simulink model "UnusedModels"  (R2015a)
settings: Solver=ode45  StartTime=0.0  StopTime=10.0  RelTol=1e-3
values from neighbouring files (symbols this model uses):
  car_params = Simulink_Car_params    [TV2016_parameters.m]
  energyLimitControl = Simulink_energyLimit    [TV2016_parameters.m]
  settings = Simulink_Settings    [TV2016_parameters.m]
  speedEstimation = Simulink_speedEst    [TV2016_parameters.m]
  tractionControl = Simulink_tc    [TV2016_parameters.m]
  yawRateControl = Simulink_yawRate    [TV2016_parameters.m]
undefined symbols (not defined in the file or in its folder): canChannel, Use_Estimated_velocity
libraries: canlib x44, CarMaker4SL x33, canmsglib x28, simulink x6
(part 1 of 4)
settings Model: Creator=Will  LastModifiedBy=Will

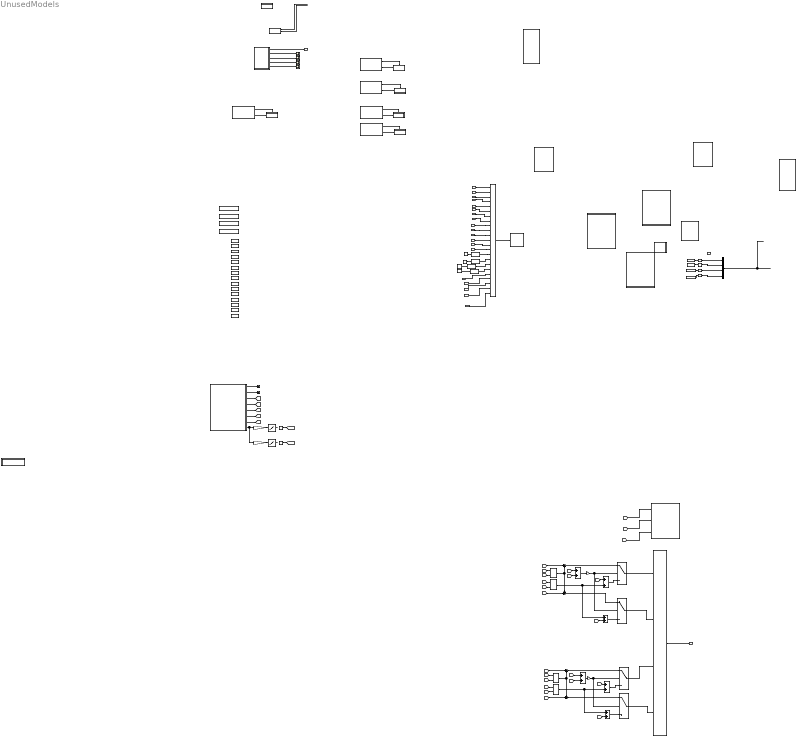
== system UnusedModels ==
  note: Tc ouput is either an increase or decrease in torque .
  "States " : Inport
  "Throttle " : Inport  Port=2
  "Brake " : Inport  Port=3
  "Steering " : Inport  Port=4
  V_x : Inport  Port=5
  V_y : Inport  Port=6
  "Fz_FL " : Inport  Port=7
  Fz_FR : Inport  Port=8
  "Fz_RL " : Inport  Port=9
  Fz_RR : Inport  Port=10
  "yawRate " : Inport  Port=11
  ay : Inport  Port=12
  ax : Inport  Port=13
  roll_angle : Inport  Port=14
  roll_rate : Inport  Port=15
  RPM_FL : Inport  Port=16
  RPM_FR : Inport  Port=17
  RPM_RL : Inport  Port=18
  RPM_RR : Inport  Port=19
  KERS_pos : Inport  Port=20
  Add{,1..5} (6 alike) : Sum
  Allocates Torque. Engineering solution : MATLAB Function  TreatAsAtomicUnit=on
  Allocates Torque. Engineering solution1 : MATLAB Function  TreatAsAtomicUnit=on
  Bus Creator : BusCreator  Inputs=23  OutDataTypeStr=Bus: SensorInputs  NonVirtualBus=on
      settings: InheritFromInputs=off
  Bus Creator1 : BusCreator  OutDataTypeStr=Bus: R_eff_i
  Bus Creator2 : BusCreator  OutDataTypeStr=Bus: Ti_lim  NonVirtualBus=on
      settings: InheritFromInputs=off
  CAN INTERFACE : Subsystem
  CAN Receive : canlib/CAN Receive  BlockHandle=13966.0022  DeviceMenu=(none)  Device=PEAK-System PCAN-USB (PCAN_USBBUS1)  ObjConstructor=canChannel('PEAK-System', 'PCAN_USBBUS1')  EnableStandardIDsFilter=off  StandardIDs=CAN_ID_INV_FL  EnableExtendedIDsFilter=off  ExtendedIDs=0  SampleTime=0.001  MsgsPerTimestep=1  StdIDsCombo=Allow only  ExtIDsCombo=Allow all  InternalFilterUpdateStatus=on
  CAN Receive1 : canlib/CAN Receive  BlockHandle=13967.002  DeviceMenu=(none)  Device=PEAK-System PCAN-USB (PCAN_USBBUS1)  ObjConstructor=canChannel('PEAK-System', 'PCAN_USBBUS1')  EnableStandardIDsFilter=off  StandardIDs=CAN_ID_INV_FR  EnableExtendedIDsFilter=off  ExtendedIDs=0  SampleTime=0.001  MsgsPerTimestep=1  StdIDsCombo=Allow only  ExtIDsCombo=Allow all  InternalFilterUpdateStatus=on
  CAN Receive2 : canlib/CAN Receive  BlockHandle=13968.0031  DeviceMenu=(none)  Device=PEAK-System PCAN-USB (PCAN_USBBUS1)  ObjConstructor=canChannel('PEAK-System', 'PCAN_USBBUS1')  EnableStandardIDsFilter=off  StandardIDs=CAN_ID_INV_RL  EnableExtendedIDsFilter=off  ExtendedIDs=0  SampleTime=0.001  MsgsPerTimestep=1  StdIDsCombo=Allow only  ExtIDsCombo=Allow all  InternalFilterUpdateStatus=on
  CAN Receive3 : canlib/CAN Receive  BlockHandle=13969.0096  DeviceMenu=(none)  Device=PEAK-System PCAN-USB (PCAN_USBBUS1)  ObjConstructor=canChannel('PEAK-System', 'PCAN_USBBUS1')  EnableStandardIDsFilter=off  StandardIDs=CAN_ID_INV_RR  EnableExtendedIDsFilter=off  ExtendedIDs=0  SampleTime=0.001  MsgsPerTimestep=1  StdIDsCombo=Allow only  ExtIDsCombo=Allow all  InternalFilterUpdateStatus=on
  CAN Receive4 : canlib/CAN Receive  BlockHandle=13970.0022  DeviceMenu=(none)  Device=PEAK-System PCAN-USB (PCAN_USBBUS1)  ObjConstructor=canChannel('PEAK-System', 'PCAN_USBBUS1')  EnableStandardIDsFilter=off  StandardIDs=[31,32,33,34]  EnableExtendedIDsFilter=off  ExtendedIDs=0  SampleTime=0.001  MsgsPerTimestep=all  StdIDsCombo=Allow only  ExtIDsCombo=Block all  InternalFilterUpdateStatus=on
  CAN Transmit : canlib/CAN Transmit  BlockHandle=14013.0021  DeviceMenu=(none)  Device=PEAK-System PCAN-USB (PCAN_USBBUS1)  ObjConstructor=canChannel('PEAK-System', 'PCAN_USBBUS1')  EnablePeriodicTransmit=on  MessagePeriod=0.005
  CAN Transmit1 : canlib/CAN Transmit  BlockHandle=14014.0021  DeviceMenu=(none)  Device=PEAK-System PCAN-USB (PCAN_USBBUS1)  ObjConstructor=canChannel('PEAK-System', 'PCAN_USBBUS1')  EnablePeriodicTransmit=on  MessagePeriod=0.005
  CAN Transmit10 : canlib/CAN Transmit  BlockHandle=14015.0021  DeviceMenu=(none)  Device=PEAK-System PCAN-USB (PCAN_USBBUS1)  ObjConstructor=canChannel('PEAK-System', 'PCAN_USBBUS1')  EnablePeriodicTransmit=on  MessagePeriod=0.005
  CAN Transmit11 : canlib/CAN Transmit  BlockHandle=14016.0021  DeviceMenu=(none)  Device=PEAK-System PCAN-USB (PCAN_USBBUS1)  ObjConstructor=canChannel('PEAK-System', 'PCAN_USBBUS1')  EnablePeriodicTransmit=on  MessagePeriod=0.005
  CAN Transmit12 : canlib/CAN Transmit  BlockHandle=14019.0021  DeviceMenu=(none)  Device=PEAK-System PCAN-USB (PCAN_USBBUS1)  ObjConstructor=canChannel('PEAK-System', 'PCAN_USBBUS1')  EnablePeriodicTransmit=on  MessagePeriod=0.005
  CAN Transmit13 : canlib/CAN Transmit  BlockHandle=14020.0021  DeviceMenu=(none)  Device=PEAK-System PCAN-USB (PCAN_USBBUS1)  ObjConstructor=canChannel('PEAK-System', 'PCAN_USBBUS1')  EnablePeriodicTransmit=on  MessagePeriod=0.005
  CAN Transmit14 : canlib/CAN Transmit  BlockHandle=14037.0066  DeviceMenu=(none)  Device=PEAK-System PCAN-USB (PCAN_USBBUS1)  ObjConstructor=canChannel('PEAK-System', 'PCAN_USBBUS1')  EnablePeriodicTransmit=on  MessagePeriod=0.005
  CAN Transmit15 : canlib/CAN Transmit  BlockHandle=14045.0049  DeviceMenu=(none)  Device=PEAK-System PCAN-USB (PCAN_USBBUS1)  ObjConstructor=canChannel('PEAK-System', 'PCAN_USBBUS1')  EnablePeriodicTransmit=on  MessagePeriod=0.005
  CAN Transmit16 : canlib/CAN Transmit  BlockHandle=14046.005  DeviceMenu=(none)  Device=PEAK-System PCAN-USB (PCAN_USBBUS1)  ObjConstructor=canChannel('PEAK-System', 'PCAN_USBBUS1')  EnablePeriodicTransmit=on  MessagePeriod=0.005
  CAN Transmit17 : canlib/CAN Transmit  BlockHandle=14047.0042  DeviceMenu=(none)  Device=PEAK-System PCAN-USB (PCAN_USBBUS1)  ObjConstructor=canChannel('PEAK-System', 'PCAN_USBBUS1')  EnablePeriodicTransmit=on  MessagePeriod=0.005
  CAN Transmit18 : canlib/CAN Transmit  BlockHandle=14048.0045  DeviceMenu=(none)  Device=PEAK-System PCAN-USB (PCAN_USBBUS1)  ObjConstructor=canChannel('PEAK-System', 'PCAN_USBBUS1')  EnablePeriodicTransmit=on  MessagePeriod=0.005
  CAN Transmit19 : canlib/CAN Transmit  BlockHandle=14206.007  DeviceMenu=(none)  Device=PEAK-System PCAN-USB (PCAN_USBBUS1)  ObjConstructor=canChannel('PEAK-System', 'PCAN_USBBUS1')  EnablePeriodicTransmit=on  MessagePeriod=0.005
  CAN Transmit3 : canlib/CAN Transmit  BlockHandle=14207.0072  DeviceMenu=(none)  Device=PEAK-System PCAN-USB (PCAN_USBBUS1)  ObjConstructor=canChannel('PEAK-System', 'PCAN_USBBUS1')  EnablePeriodicTransmit=on  MessagePeriod=0.005
  CAN Transmit4 : canlib/CAN Transmit  BlockHandle=14208.0072  DeviceMenu=(none)  Device=PEAK-System PCAN-USB (PCAN_USBBUS1)  ObjConstructor=canChannel('PEAK-System', 'PCAN_USBBUS1')  EnablePeriodicTransmit=on  MessagePeriod=0.005
  CAN Transmit5 : canlib/CAN Transmit  BlockHandle=14314.0065  DeviceMenu=(none)  Device=PEAK-System PCAN-USB (PCAN_USBBUS1)  ObjConstructor=canChannel('PEAK-System', 'PCAN_USBBUS1')  EnablePeriodicTransmit=on  MessagePeriod=0.005
  CAN Transmit6 : canlib/CAN Transmit  BlockHandle=14316.0067  DeviceMenu=(none)  Device=PEAK-System PCAN-USB (PCAN_USBBUS1)  ObjConstructor=canChannel('PEAK-System', 'PCAN_USBBUS1')  EnablePeriodicTransmit=off  MessagePeriod=0.005
  CAN Transmit7 : canlib/CAN Transmit  BlockHandle=14318.0065  DeviceMenu=(none)  Device=PEAK-System PCAN-USB (PCAN_USBBUS1)  ObjConstructor=canChannel('PEAK-System', 'PCAN_USBBUS1')  EnablePeriodicTransmit=on  MessagePeriod=0.005
  CAN Transmit8 : canlib/CAN Transmit  BlockHandle=14320.0065  DeviceMenu=(none)  Device=PEAK-System PCAN-USB (PCAN_USBBUS1)  ObjConstructor=canChannel('PEAK-System', 'PCAN_USBBUS1')  EnablePeriodicTransmit=on  MessagePeriod=0.005
  CAN Transmit9 : canlib/CAN Transmit  BlockHandle=14345.005  DeviceMenu=(none)  Device=PEAK-System PCAN-USB (PCAN_USBBUS1)  ObjConstructor=canChannel('PEAK-System', 'PCAN_USBBUS1')  EnablePeriodicTransmit=on  MessagePeriod=0.005
  Coasting KERS at 0 torque request : Subsystem
  Constant : Constant  Value=tractionControl.Kp
  Constant{1..4} (4 alike) : Constant
  Constant5 : Constant  Value=tractionControl.Ki
  Data Type Conversion{,1..6,12} (8 alike) : DataTypeConversion  OutDataTypeStr=single
  Energy limit Torque Reduction Controller : Subsystem
  "Estimations " : Subsystem  SystemSampleTime=settings.control_system_sample_time
  Function-Call Subsystem : Subsystem  TreatAsAtomicUnit=on
  Function-Call Subsystem1 : Subsystem  TreatAsAtomicUnit=on
  Function-Call Subsystem2 : Subsystem  TreatAsAtomicUnit=on
  Function-Call Subsystem3 : Subsystem  TreatAsAtomicUnit=on
  Function-Call Subsystem4 : Subsystem  TreatAsAtomicUnit=on
  FzCalcRaw : Scope
      settings: ShowLegends=on  TimeRange=0.5129057337220599  YMin=982.0067255187187  YMax=982.99982331966  SaveName=ScopeData4
  FzEstCoupledKalmanFilters : MATLAB Function  TreatAsAtomicUnit=on
  Fz_Estimation : Subsystem  TreatAsAtomicUnit=on
  Gain : Gain  Gain=single(3.6)
  Gain1 : Gain  Gain=-1
  Gain2 : Gain  Gain=single(3.6)
  Gain3 : Gain  Gain=-1
  Ki Loopup : Lookup_n-D  NumberOfTableDimensions=1  BreakpointsForDimension1=[0 10]  Table="[tractionControl.Ki_start  tractionControl.Ki_end]*tractionControl.Ki_scaling"  ExtrapMethod=Clip  UseLastTableValue=on  InternalRulePriority=Speed  RndMeth=Simplest  InputSameDT=on
  Kp Lookup : Lookup_n-D  NumberOfTableDimensions=1  BreakpointsForDimension1="[0  10]"  Table="[tractionControl.Kp_start  tractionControl.Kp_end]*tractionControl.Kp_scaling"  ExtrapMethod=Clip  UseLastTableValue=on  InternalRulePriority=Speed  RndMeth=Simplest  InputSameDT=on
  MATLAB Function : MATLAB Function  TreatAsAtomicUnit=on
  Min : MinMax  Inputs=2
  Min1 : MinMax  Function=max  Inputs=2
  Min4 : MinMax  Inputs=2
  Min5 : MinMax  Function=max  Inputs=2
  Read CM Dict10 : CarMaker4SL/Read CM Dict  xname=Car.WFR.Radius  xsync=off
  Read CM Dict11 : CarMaker4SL/Read CM Dict  xname=Car.WRR.Radius  xsync=off
  Read CM Dict12 : CarMaker4SL/Read CM Dict  xname=Car.WRL.Radius  xsync=off
  Read CM Dict9 : CarMaker4SL/Read CM Dict  xname=Car.WFL.Radius  xsync=off
  SimpleTv : Subsystem
  Slip rate Both3 : Subsystem
  Slip rate Both6 : Subsystem
  Slip rate FL : Subsystem
  Slip rate FL1 : Subsystem
  Slip ratio : MATLAB Function  TreatAsAtomicUnit=on
  Sum : Sum  Inputs=|++
  Sum1 : Sum  Inputs=++|
  Sum2 : Sum  Inputs=|++
  Sum4 : Sum  Inputs=++|
  Switch : Switch  Criteria=u2 > Threshold
  Switch1 : Switch  Criteria=u2 > Threshold  Threshold=0.0001
  Switch4 : Switch  Criteria=u2 > Threshold
  Switch5 : Switch  Criteria=u2 > Threshold
  Terminator : Terminator
  Terminator1 : Terminator
  "deltaFz " : Scope
      settings: ShowLegends=on  TimeRange=10  YMin=-650  YMax=50  SaveName=ScopeData5
  lateral : Scope
      settings: ShowLegends=on  TimeRange=1.971383147853736  YMin=574.5308310991956  YMax=1245.308310991957  SaveName=ScopeData8
  speedEstimate : Subsystem  TreatAsAtomicUnit=on
  vertialest : Scope
      settings: ShowLegends=on  TimeRange=2.029755579171094  YMin=-50  YMax=950  SaveName=ScopeData10
  Ti_SR : Outport
  Fz_Kalman_est : Outport  Port=2
  tag scope: SR_RL=global, SR_RR=global
  wires:
  Read CM Dict9/1 -> Data Type Conversion/1
  Read CM Dict11/1 -> Data Type Conversion2/1
  Read CM Dict12/1 -> Data Type Conversion3/1
  Read CM Dict10/1 -> Data Type Conversion1/1
  Data Type Conversion3/1 -> Bus Creator1/4  "R_RL"
  Data Type Conversion1/1 -> Bus Creator1/2  "R_FR"
  Data Type Conversion2/1 -> Bus Creator1/3  "R_RR"
  Data Type Conversion/1 -> Bus Creator1/1  "R_FL"
  Bus Creator1/1 -> ?
  "Brake "/1 -> Bus Creator/9  "Input_brake"
  "Steering "/1 -> Bus Creator/10  "Input_steering"
  Fz_RR/1 -> Bus Creator/5  "Input_Fz_RR"
  "Fz_RL "/1 -> Bus Creator/4  "Input_Fz_RL"
  "Fz_FL "/1 -> Bus Creator/2  "Input_Fz_FL"
  Fz_FR/1 -> Bus Creator/3  "Input_Fz_FR"
  V_y/1 -> Bus Creator/7  "V_y"
  V_x/1 -> Bus Creator/6  "V_x"
  "yawRate "/1 -> Bus Creator/1  "r"
  "Throttle "/1 -> Bus Creator/8  "Input_throttle"
  ay/1 -> Bus Creator/11  "ay"
  ax/1 -> Bus Creator/12  "ax"
  roll_angle/1 -> Bus Creator/13  "roll_angle"
  roll_rate/1 -> Bus Creator/14  "roll_rate"
  Constant1/1 -> Data Type Conversion12/1
  Data Type Conversion12/1 -> Bus Creator/15  "d_def_FL"
  Constant2/1 -> Data Type Conversion4/1
  Data Type Conversion4/1 -> Bus Creator/16  "d_def_FR"
  Constant3/1 -> Data Type Conversion5/1
  Data Type Conversion5/1 -> Bus Creator/17  "d_def_RL"
  Constant4/1 -> Data Type Conversion6/1
  Data Type Conversion6/1 -> Bus Creator/18  "d_def_RR"
  RPM_FL/1 -> Bus Creator/19  "RPM_FL"
  RPM_FR/1 -> Bus Creator/20  "RPM_FR"
  RPM_RL/1 -> Bus Creator/21  "RPM_RL"
  RPM_RR/1 -> Bus Creator/22  "RPM_RR"
  KERS_pos/1 -> Bus Creator/23  "KERS_pos"
  Bus Creator/1 -> "Estimations "/1("SensorInputs ")
  CAN Receive/2 -> Function-Call Subsystem/1(CAN_MSG)
  CAN Receive/1 -> Function-Call Subsystem/Trigger
  CAN Receive1/2 -> Function-Call Subsystem1/1(CAN_MSG)
  CAN Receive1/1 -> Function-Call Subsystem1/Trigger
  CAN Receive2/2 -> Function-Call Subsystem2/1(CAN_MSG)
  CAN Receive2/1 -> Function-Call Subsystem2/Trigger
  CAN Receive3/2 -> Function-Call Subsystem3/1(CAN_MSG)
  CAN Receive3/1 -> Function-Call Subsystem3/Trigger
  CAN Receive4/2 -> Function-Call Subsystem4/1(CAN_MSG)
  CAN Receive4/1 -> Function-Call Subsystem4/Trigger
  [Ti_RR] -> Slip rate Both6/3(Ti_ref)
  [SR_ref] -> Slip rate Both6/1(SR_ref)
  [SR_RR] -> Slip rate Both6/2(SR)
  Add4/1 -> Gain1/1
  Min/1 -> Sum1/1, Sum/2
  [Ti_FR] -> Sum1/2  "FR"
  Min1/1 -> Add1/1, Add/2
  Add1/1 -> Switch1/3
  [Ti_FL] -> Sum/1
  [Ti_FL] -> Add/1
  Add/1 -> Switch/3
  [TC_FL] -> Min/1
  [TC_FR] -> Min/2
  [TC_FR] -> Min1/2
  [TC_FL] -> Min1/1
  [Ti_FR] -> Add1/2
  [TC_FR] -> Add4/2
  [TC_FL] -> Add4/1
  Switch1/1 -> Bus Creator2/2  "FR"
  Switch/1 -> Bus Creator2/1  "FL"
  Gain3/1 -> Switch5/2, Switch4/2
  Min4/1 -> Sum4/1, Sum2/2
  Sum2/1 -> Switch4/1
  [Ti_RR] -> Sum4/2  "FR"
  Sum4/1 -> Switch5/1
  Min5/1 -> Add3/1, Add2/2
  Add3/1 -> Switch5/3
  [Ti_RL] -> Sum2/1
  [Ti_RL] -> Add2/1
  Add2/1 -> Switch4/3
  [TC_RL] -> Min4/1
  [TC_RR] -> Min4/2
  [TC_RR] -> Min5/2
  [TC_RL] -> Min5/1
  [Ti_RR] -> Add3/2
  [TC_RR] -> Add5/2
  [TC_RL] -> Add5/1
  Switch5/1 -> Bus Creator2/4  "RR"
  Switch4/1 -> Bus Creator2/3  "RL"
  Bus Creator2/1 -> Ti_SR/1
  Gain1/1 -> Switch1/2, Switch/2
  Add5/1 -> Gain3/1
  Sum/1 -> Switch/1
  Sum1/1 -> Switch1/1
  Slip ratio/3(SR_ref) -> [SR_ref]
  Slip ratio/4(SR_FL) -> [SR_FL]
  Slip ratio/5(SR_FR) -> [SR_FR]
  Slip ratio/6(SR_RL) -> [SR_RL]
  Slip ratio/7(SR_RR) -> [SR_RR]
  Slip ratio/2(SR_Ki) -> Terminator1/1
  Slip ratio/1(SR_Kp) -> Terminator/1
  Slip ratio/8(speed) -> Gain/1, Gain2/1
  Kp Lookup/1 -> ?
  Ki Loopup/1 -> ?
  Gain/1 -> Kp Lookup/1
  Gain2/1 -> Ki Loopup/1
  Constant5/1 -> [SR_Ki]
  Constant/1 -> [SR_Kp]
  FzEstCoupledKalmanFilters/2(x_out) -> lateral/1
  FzEstCoupledKalmanFilters/3(xv_out) -> vertialest/1
  FzEstCoupledKalmanFilters/4(FZ) -> FzCalcRaw/1
  FzEstCoupledKalmanFilters/5(delta_Fzl) -> "deltaFz "/1
  FzEstCoupledKalmanFilters/1(normalForces) -> Fz_Kalman_est/1
  ? -> Coasting KERS at 0 torque request/1(states)
  Coasting KERS at 0 torque request/1(active) -> ?
  Coasting KERS at 0 torque request/2(Ti_coast) -> ?

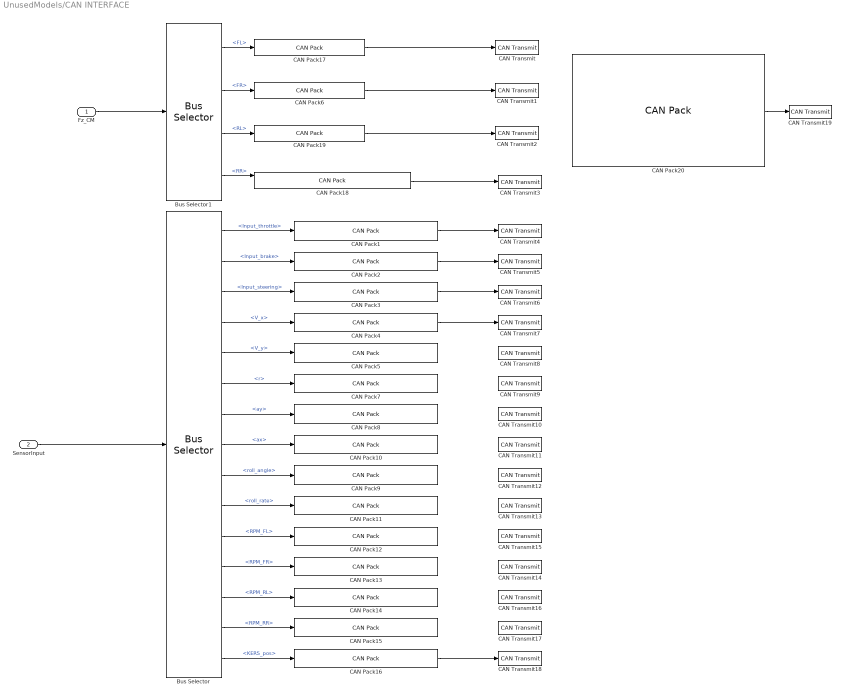
== system UnusedModels/CAN INTERFACE ==
  Fz_CM : Inport
  SensorInput : Inport  Port=2
  Bus Selector : BusSelector  OutputSignals=Input_throttle,Input_brake,Input_steering,V_x,V_y,r,ay,ax,roll_angle,roll_rate,RPM_FL,RPM_FR,RPM_RL,RPM_RR,KERS_pos
  Bus Selector1 : BusSelector  OutputSignals=FL,FR,RL,RR
  CAN Pack1 : canmsglib/CAN Pack  MsgList=(none)  MsgName=gas  MsgIDType=Standard (11-bit identifier)  MsgIdentifier=CAN_ID_GAS  MsgLength=8  SignalInfo=gas$0$32$1$3$1$0$1$0$-Inf$Inf$#  NSignals=1  StartBits=str2num('[int32(0)]')  SignalSizes=str2num('[int32(32)]')  ByteOrders=str2num('[int32(1)]')  DataTypes=str2num('[int32(3)]')  MultiplexTypes=str2num('[int32(1)]')  MultiplexValues=str2num('[double(0)]')  Factors=str2num('[double(1)]')  Offsets=str2num('[double(0)]')  Minimums=str2num('[double(-Inf)]')  Maximums=str2num('[double(Inf)]')  Remote=off
      settings: DataFormat=manually specified signals
  CAN Pack10 : canmsglib/CAN Pack  MsgList=(none)  MsgName=ax  MsgIDType=Standard (11-bit identifier)  MsgIdentifier=CAN_ID_AX  MsgLength=4  SignalInfo=ax$0$32$1$3$1$0$1$0$-Inf$Inf$#  NSignals=1  StartBits=str2num('[int32(0)]')  SignalSizes=str2num('[int32(32)]')  ByteOrders=str2num('[int32(1)]')  DataTypes=str2num('[int32(3)]')  MultiplexTypes=str2num('[int32(1)]')  MultiplexValues=str2num('[double(0)]')  Factors=str2num('[double(1)]')  Offsets=str2num('[double(0)]')  Minimums=str2num('[double(-Inf)]')  Maximums=str2num('[double(Inf)]')  Remote=off
      settings: DataFormat=manually specified signals
  CAN Pack11 : canmsglib/CAN Pack  MsgList=(none)  MsgName=roll_rate  MsgIDType=Standard (11-bit identifier)  MsgIdentifier=CAN_ID_ROLL_RATE  MsgLength=4  SignalInfo=roll_rate$0$32$1$3$1$0$1$0$-Inf$Inf$#  NSignals=1  StartBits=str2num('[int32(0)]')  SignalSizes=str2num('[int32(32)]')  ByteOrders=str2num('[int32(1)]')  DataTypes=str2num('[int32(3)]')  MultiplexTypes=str2num('[int32(1)]')  MultiplexValues=str2num('[double(0)]')  Factors=str2num('[double(1)]')  Offsets=str2num('[double(0)]')  Minimums=str2num('[double(-Inf)]')  Maximums=str2num('[double(Inf)]')  Remote=off
      settings: DataFormat=manually specified signals
  CAN Pack12 : canmsglib/CAN Pack  MsgList=(none)  MsgName=RPM_FL  MsgIDType=Standard (11-bit identifier)  MsgIdentifier=CAN_ID_RPM_FL  MsgLength=4  SignalInfo=RPM_FL$0$32$1$3$1$0$1$0$-Inf$Inf$#  NSignals=1  StartBits=str2num('[int32(0)]')  SignalSizes=str2num('[int32(32)]')  ByteOrders=str2num('[int32(1)]')  DataTypes=str2num('[int32(3)]')  MultiplexTypes=str2num('[int32(1)]')  MultiplexValues=str2num('[double(0)]')  Factors=str2num('[double(1)]')  Offsets=str2num('[double(0)]')  Minimums=str2num('[double(-Inf)]')  Maximums=str2num('[double(Inf)]')  Remote=off
      settings: DataFormat=manually specified signals
  CAN Pack13 : canmsglib/CAN Pack  MsgList=(none)  MsgName=RPM_FR  MsgIDType=Standard (11-bit identifier)  MsgIdentifier=CAN_ID_RPM_FR  MsgLength=4  SignalInfo=RPM_FR$0$32$1$3$1$0$1$0$-Inf$Inf$#  NSignals=1  StartBits=str2num('[int32(0)]')  SignalSizes=str2num('[int32(32)]')  ByteOrders=str2num('[int32(1)]')  DataTypes=str2num('[int32(3)]')  MultiplexTypes=str2num('[int32(1)]')  MultiplexValues=str2num('[double(0)]')  Factors=str2num('[double(1)]')  Offsets=str2num('[double(0)]')  Minimums=str2num('[double(-Inf)]')  Maximums=str2num('[double(Inf)]')  Remote=off
      settings: DataFormat=manually specified signals
  CAN Pack14 : canmsglib/CAN Pack  MsgList=(none)  MsgName=RPM_RL  MsgIDType=Standard (11-bit identifier)  MsgIdentifier=CAN_ID_RPM_RL  MsgLength=4  SignalInfo=RPM_RL$0$32$1$3$1$0$1$0$-Inf$Inf$#  NSignals=1  StartBits=str2num('[int32(0)]')  SignalSizes=str2num('[int32(32)]')  ByteOrders=str2num('[int32(1)]')  DataTypes=str2num('[int32(3)]')  MultiplexTypes=str2num('[int32(1)]')  MultiplexValues=str2num('[double(0)]')  Factors=str2num('[double(1)]')  Offsets=str2num('[double(0)]')  Minimums=str2num('[double(-Inf)]')  Maximums=str2num('[double(Inf)]')  Remote=off
      settings: DataFormat=manually specified signals
  CAN Pack15 : canmsglib/CAN Pack  MsgList=(none)  MsgName=RPM_RR  MsgIDType=Standard (11-bit identifier)  MsgIdentifier=CAN_ID_RPM_RR  MsgLength=4  SignalInfo=RPM_RR$0$32$1$3$1$0$1$0$-Inf$Inf$#  NSignals=1  StartBits=str2num('[int32(0)]')  SignalSizes=str2num('[int32(32)]')  ByteOrders=str2num('[int32(1)]')  DataTypes=str2num('[int32(3)]')  MultiplexTypes=str2num('[int32(1)]')  MultiplexValues=str2num('[double(0)]')  Factors=str2num('[double(1)]')  Offsets=str2num('[double(0)]')  Minimums=str2num('[double(-Inf)]')  Maximums=str2num('[double(Inf)]')  Remote=off
      settings: DataFormat=manually specified signals
  CAN Pack16 : canmsglib/CAN Pack  MsgList=(none)  MsgName=KERS_POS  MsgIDType=Standard (11-bit identifier)  MsgIdentifier=CAN_ID_KERS_POS  MsgLength=4  SignalInfo=KERS_POS$0$32$1$3$1$0$1$0$-Inf$Inf$#  NSignals=1  StartBits=str2num('[int32(0)]')  SignalSizes=str2num('[int32(32)]')  ByteOrders=str2num('[int32(1)]')  DataTypes=str2num('[int32(3)]')  MultiplexTypes=str2num('[int32(1)]')  MultiplexValues=str2num('[double(0)]')  Factors=str2num('[double(1)]')  Offsets=str2num('[double(0)]')  Minimums=str2num('[double(-Inf)]')  Maximums=str2num('[double(Inf)]')  Remote=off
      settings: DataFormat=manually specified signals
  CAN Pack17 : canmsglib/CAN Pack  MsgList=(none)  MsgName=Fz_FL  MsgIDType=Standard (11-bit identifier)  MsgIdentifier=CAN_ID_FZ_FL  MsgLength=4  SignalInfo=Fz_FL$0$32$1$3$1$0$1$0$-Inf$Inf$#  NSignals=1  StartBits=str2num('[int32(0)]')  SignalSizes=str2num('[int32(32)]')  ByteOrders=str2num('[int32(1)]')  DataTypes=str2num('[int32(3)]')  MultiplexTypes=str2num('[int32(1)]')  MultiplexValues=str2num('[double(0)]')  Factors=str2num('[double(1)]')  Offsets=str2num('[double(0)]')  Minimums=str2num('[double(-Inf)]')  Maximums=str2num('[double(Inf)]')  Remote=off
      settings: DataFormat=manually specified signals
  CAN Pack18 : canmsglib/CAN Pack  MsgList=(none)  MsgName=Fz_RR  MsgIDType=Standard (11-bit identifier)  MsgIdentifier=CAN_ID_FZ_RR  MsgLength=8  SignalInfo=Fz_RR$0$32$1$3$1$0$1$0$-Inf$Inf$#Signal2$32$32$1$1$1$0$1$0$-Inf$Inf$#  NSignals=2  StartBits=str2num('[int32(0);int32(32)]')  SignalSizes=str2num('[int32(32);int32(32)]')  ByteOrders=str2num('[int32(1);int32(1)]')  DataTypes=str2num('[int32(3);int32(1)]')  MultiplexTypes=str2num('[int32(1);int32(1)]')  MultiplexValues=str2num('[double(0);double(0)]')  Factors=str2num('[double(1);double(1)]')  Offsets=str2num('[double(0);double(0)]')  Minimums=str2num('[double(-Inf);double(-Inf)]')  Maximums=str2num('[double(Inf);double(Inf)]')  Remote=off
      settings: DataFormat=manually specified signals
  CAN Pack19 : canmsglib/CAN Pack  MsgList=(none)  MsgName=Fz_RL  MsgIDType=Standard (11-bit identifier)  MsgIdentifier=CAN_ID_FZ_RL  MsgLength=4  SignalInfo=Fz_RL$0$32$1$3$1$0$1$0$-Inf$Inf$#  NSignals=1  StartBits=str2num('[int32(0)]')  SignalSizes=str2num('[int32(32)]')  ByteOrders=str2num('[int32(1)]')  DataTypes=str2num('[int32(3)]')  MultiplexTypes=str2num('[int32(1)]')  MultiplexValues=str2num('[double(0)]')  Factors=str2num('[double(1)]')  Offsets=str2num('[double(0)]')  Minimums=str2num('[double(-Inf)]')  Maximums=str2num('[double(Inf)]')  Remote=off
      settings: DataFormat=manually specified signals
  CAN Pack2 : canmsglib/CAN Pack  MsgList=(none)  MsgName=brake  MsgIDType=Standard (11-bit identifier)  MsgIdentifier=CAN_ID_BRAKE  MsgLength=8  SignalInfo=brake$0$32$1$3$1$0$1$0$-Inf$Inf$#  NSignals=1  StartBits=str2num('[int32(0)]')  SignalSizes=str2num('[int32(32)]')  ByteOrders=str2num('[int32(1)]')  DataTypes=str2num('[int32(3)]')  MultiplexTypes=str2num('[int32(1)]')  MultiplexValues=str2num('[double(0)]')  Factors=str2num('[double(1)]')  Offsets=str2num('[double(0)]')  Minimums=str2num('[double(-Inf)]')  Maximums=str2num('[double(Inf)]')  Remote=off
      settings: DataFormat=manually specified signals
  CAN Pack20 : canmsglib/CAN Pack  MsgList=(none)  MsgName=Fz  MsgIDType=Standard (11-bit identifier)  MsgIdentifier=CAN_ID_FZ  MsgLength=8  SignalInfo=Fz_FL$0$16$1$2$1$0$1$0$-Inf$Inf$#Fz_FR$16$16$1$2$1$0$1$0$-Inf$Inf$#Fz_RL$32$16$1$2$1$0$1$0$-Inf$Inf$#Fz_RR$48$16$1$2$1$0$1$0$-Inf$Inf$#  NSignals=4  StartBits=str2num('[int32(0);int32(16);int32(32);int32(48)]')  SignalSizes=str2num('[int32(16);int32(16);int32(16);int32(16)]')  ByteOrders=str2num('[int32(1);int32(1);int32(1);int32(1)]')  DataTypes=str2num('[int32(2);int32(2);int32(2);int32(2)]')  MultiplexTypes=str2num('[int32(1);int32(1);int32(1);int32(1)]')  MultiplexValues=str2num('[double(0);double(0);double(0);double(0)]')  Factors=str2num('[double(1);double(1);double(1);double(1)]')  Offsets=str2num('[double(0);double(0);double(0);double(0)]')  Minimums=str2num('[double(-Inf);double(-Inf);double(-Inf);double(-Inf)]')  Maximums=str2num('[double(Inf);double(Inf);double(Inf);double(Inf)]')  Remote=off
      settings: DataFormat=manually specified signals
  CAN Pack3 : canmsglib/CAN Pack  MsgList=(none)  MsgName=steering  MsgIDType=Standard (11-bit identifier)  MsgIdentifier=CAN_ID_STEERING  MsgLength=8  SignalInfo=steering$0$32$1$3$1$0$1$0$-Inf$Inf$#  NSignals=1  StartBits=str2num('[int32(0)]')  SignalSizes=str2num('[int32(32)]')  ByteOrders=str2num('[int32(1)]')  DataTypes=str2num('[int32(3)]')  MultiplexTypes=str2num('[int32(1)]')  MultiplexValues=str2num('[double(0)]')  Factors=str2num('[double(1)]')  Offsets=str2num('[double(0)]')  Minimums=str2num('[double(-Inf)]')  Maximums=str2num('[double(Inf)]')  Remote=off
      settings: DataFormat=manually specified signals
  CAN Pack4 : canmsglib/CAN Pack  MsgList=(none)  MsgName=vx  MsgIDType=Standard (11-bit identifier)  MsgIdentifier=CAN_ID_VX  MsgLength=4  SignalInfo=vx$0$32$1$3$1$0$1$0$-Inf$Inf$#  NSignals=1  StartBits=str2num('[int32(0)]')  SignalSizes=str2num('[int32(32)]')  ByteOrders=str2num('[int32(1)]')  DataTypes=str2num('[int32(3)]')  MultiplexTypes=str2num('[int32(1)]')  MultiplexValues=str2num('[double(0)]')  Factors=str2num('[double(1)]')  Offsets=str2num('[double(0)]')  Minimums=str2num('[double(-Inf)]')  Maximums=str2num('[double(Inf)]')  Remote=off
      settings: DataFormat=manually specified signals
  CAN Pack5 : canmsglib/CAN Pack  MsgList=(none)  MsgName=vy  MsgIDType=Standard (11-bit identifier)  MsgIdentifier=CAN_ID_VY  MsgLength=4  SignalInfo=vy$0$32$1$3$1$0$1$0$-Inf$Inf$#  NSignals=1  StartBits=str2num('[int32(0)]')  SignalSizes=str2num('[int32(32)]')  ByteOrders=str2num('[int32(1)]')  DataTypes=str2num('[int32(3)]')  MultiplexTypes=str2num('[int32(1)]')  MultiplexValues=str2num('[double(0)]')  Factors=str2num('[double(1)]')  Offsets=str2num('[double(0)]')  Minimums=str2num('[double(-Inf)]')  Maximums=str2num('[double(Inf)]')  Remote=off
      settings: DataFormat=manually specified signals
  CAN Pack6 : canmsglib/CAN Pack  MsgList=(none)  MsgName=Fz_FR  MsgIDType=Standard (11-bit identifier)  MsgIdentifier=CAN_ID_FZ_FR  MsgLength=4  SignalInfo=Fz_FR$0$32$1$3$1$0$1$0$-Inf$Inf$#  NSignals=1  StartBits=str2num('[int32(0)]')  SignalSizes=str2num('[int32(32)]')  ByteOrders=str2num('[int32(1)]')  DataTypes=str2num('[int32(3)]')  MultiplexTypes=str2num('[int32(1)]')  MultiplexValues=str2num('[double(0)]')  Factors=str2num('[double(1)]')  Offsets=str2num('[double(0)]')  Minimums=str2num('[double(-Inf)]')  Maximums=str2num('[double(Inf)]')  Remote=off
      settings: DataFormat=manually specified signals
  CAN Pack7 : canmsglib/CAN Pack  MsgList=(none)  MsgName=r  MsgIDType=Standard (11-bit identifier)  MsgIdentifier=CAN_ID_YAW_RATE  MsgLength=4  SignalInfo=r$0$32$1$3$1$0$1$0$-Inf$Inf$#  NSignals=1  StartBits=str2num('[int32(0)]')  SignalSizes=str2num('[int32(32)]')  ByteOrders=str2num('[int32(1)]')  DataTypes=str2num('[int32(3)]')  MultiplexTypes=str2num('[int32(1)]')  MultiplexValues=str2num('[double(0)]')  Factors=str2num('[double(1)]')  Offsets=str2num('[double(0)]')  Minimums=str2num('[double(-Inf)]')  Maximums=str2num('[double(Inf)]')  Remote=off
      settings: DataFormat=manually specified signals
  CAN Pack8 : canmsglib/CAN Pack  MsgList=(none)  MsgName=ay  MsgIDType=Standard (11-bit identifier)  MsgIdentifier=CAN_ID_AY  MsgLength=4  SignalInfo=ay$0$32$1$3$1$0$1$0$-Inf$Inf$#  NSignals=1  StartBits=str2num('[int32(0)]')  SignalSizes=str2num('[int32(32)]')  ByteOrders=str2num('[int32(1)]')  DataTypes=str2num('[int32(3)]')  MultiplexTypes=str2num('[int32(1)]')  MultiplexValues=str2num('[double(0)]')  Factors=str2num('[double(1)]')  Offsets=str2num('[double(0)]')  Minimums=str2num('[double(-Inf)]')  Maximums=str2num('[double(Inf)]')  Remote=off
      settings: DataFormat=manually specified signals
  CAN Pack9 : canmsglib/CAN Pack  MsgList=(none)  MsgName=roll_angle  MsgIDType=Standard (11-bit identifier)  MsgIdentifier=CAN_ID_ROLL_ANGLE  MsgLength=4  SignalInfo=roll_angle$0$32$1$3$1$0$1$0$-Inf$Inf$#  NSignals=1  StartBits=str2num('[int32(0)]')  SignalSizes=str2num('[int32(32)]')  ByteOrders=str2num('[int32(1)]')  DataTypes=str2num('[int32(3)]')  MultiplexTypes=str2num('[int32(1)]')  MultiplexValues=str2num('[double(0)]')  Factors=str2num('[double(1)]')  Offsets=str2num('[double(0)]')  Minimums=str2num('[double(-Inf)]')  Maximums=str2num('[double(Inf)]')  Remote=off
      settings: DataFormat=manually specified signals
  CAN Transmit : canlib/CAN Transmit  BlockHandle=35.0001  DeviceMenu=PEAK-System PCAN-USB (PCAN_USBBUS1)  Device=PEAK-System PCAN-USB (PCAN_USBBUS1)  ObjConstructor=canChannel('PEAK-System', 'PCAN_USBBUS1')  EnablePeriodicTransmit=on  MessagePeriod=0.005
  CAN Transmit1 : canlib/CAN Transmit  BlockHandle=4653.0004  DeviceMenu=PEAK-System PCAN-USB (PCAN_USBBUS1)  Device=PEAK-System PCAN-USB (PCAN_USBBUS1)  ObjConstructor=canChannel('PEAK-System', 'PCAN_USBBUS1')  EnablePeriodicTransmit=on  MessagePeriod=0.005
  CAN Transmit10 : canlib/CAN Transmit  BlockHandle=7080.0005  DeviceMenu=PEAK-System PCAN-USB (PCAN_USBBUS1)  Device=PEAK-System PCAN-USB (PCAN_USBBUS1)  ObjConstructor=canChannel('PEAK-System', 'PCAN_USBBUS1')  EnablePeriodicTransmit=on  MessagePeriod=0.005
  CAN Transmit11 : canlib/CAN Transmit  BlockHandle=7090.0002  DeviceMenu=PEAK-System PCAN-USB (PCAN_USBBUS1)  Device=PEAK-System PCAN-USB (PCAN_USBBUS1)  ObjConstructor=canChannel('PEAK-System', 'PCAN_USBBUS1')  EnablePeriodicTransmit=on  MessagePeriod=0.005
  CAN Transmit12 : canlib/CAN Transmit  BlockHandle=7096.0002  DeviceMenu=PEAK-System PCAN-USB (PCAN_USBBUS1)  Device=PEAK-System PCAN-USB (PCAN_USBBUS1)  ObjConstructor=canChannel('PEAK-System', 'PCAN_USBBUS1')  EnablePeriodicTransmit=on  MessagePeriod=0.005
  CAN Transmit13 : canlib/CAN Transmit  BlockHandle=7100.0002  DeviceMenu=PEAK-System PCAN-USB (PCAN_USBBUS1)  Device=PEAK-System PCAN-USB (PCAN_USBBUS1)  ObjConstructor=canChannel('PEAK-System', 'PCAN_USBBUS1')  EnablePeriodicTransmit=on  MessagePeriod=0.005
  CAN Transmit14 : canlib/CAN Transmit  BlockHandle=7193.0006  DeviceMenu=PEAK-System PCAN-USB (PCAN_USBBUS1)  Device=PEAK-System PCAN-USB (PCAN_USBBUS1)  ObjConstructor=canChannel('PEAK-System', 'PCAN_USBBUS1')  EnablePeriodicTransmit=on  MessagePeriod=0.005
  CAN Transmit15 : canlib/CAN Transmit  BlockHandle=7553.0004  DeviceMenu=PEAK-System PCAN-USB (PCAN_USBBUS1)  Device=PEAK-System PCAN-USB (PCAN_USBBUS1)  ObjConstructor=canChannel('PEAK-System', 'PCAN_USBBUS1')  EnablePeriodicTransmit=on  MessagePeriod=0.005
  CAN Transmit16 : canlib/CAN Transmit  BlockHandle=7557.0006  DeviceMenu=PEAK-System PCAN-USB (PCAN_USBBUS1)  Device=PEAK-System PCAN-USB (PCAN_USBBUS1)  ObjConstructor=canChannel('PEAK-System', 'PCAN_USBBUS1')  EnablePeriodicTransmit=on  MessagePeriod=0.005
  CAN Transmit17 : canlib/CAN Transmit  BlockHandle=7560.0004  DeviceMenu=PEAK-System PCAN-USB (PCAN_USBBUS1)  Device=PEAK-System PCAN-USB (PCAN_USBBUS1)  ObjConstructor=canChannel('PEAK-System', 'PCAN_USBBUS1')  EnablePeriodicTransmit=on  MessagePeriod=0.005
  CAN Transmit18 : canlib/CAN Transmit  BlockHandle=7563.0004  DeviceMenu=PEAK-System PCAN-USB (PCAN_USBBUS1)  Device=PEAK-System PCAN-USB (PCAN_USBBUS1)  ObjConstructor=canChannel('PEAK-System', 'PCAN_USBBUS1')  EnablePeriodicTransmit=on  MessagePeriod=0.005
  CAN Transmit19 : canlib/CAN Transmit  BlockHandle=42.0002  DeviceMenu=PEAK-System PCAN-USB (PCAN_USBBUS1)  Device=PEAK-System PCAN-USB (PCAN_USBBUS1)  ObjConstructor=canChannel('PEAK-System', 'PCAN_USBBUS1')  EnablePeriodicTransmit=on  MessagePeriod=0.005
  CAN Transmit2 : canlib/CAN Transmit  BlockHandle=4711.0004  DeviceMenu=PEAK-System PCAN-USB (PCAN_USBBUS1)  Device=PEAK-System PCAN-USB (PCAN_USBBUS1)  ObjConstructor=canChannel('PEAK-System', 'PCAN_USBBUS1')  EnablePeriodicTransmit=on  MessagePeriod=0.005
  CAN Transmit3 : canlib/CAN Transmit  BlockHandle=5058.0006  DeviceMenu=PEAK-System PCAN-USB (PCAN_USBBUS1)  Device=PEAK-System PCAN-USB (PCAN_USBBUS1)  ObjConstructor=canChannel('PEAK-System', 'PCAN_USBBUS1')  EnablePeriodicTransmit=on  MessagePeriod=0.005
  CAN Transmit4 : canlib/CAN Transmit  BlockHandle=5623.0006  DeviceMenu=PEAK-System PCAN-USB (PCAN_USBBUS1)  Device=PEAK-System PCAN-USB (PCAN_USBBUS1)  ObjConstructor=canChannel('PEAK-System', 'PCAN_USBBUS1')  EnablePeriodicTransmit=on  MessagePeriod=0.005
  CAN Transmit5 : canlib/CAN Transmit  BlockHandle=5677.0004  DeviceMenu=PEAK-System PCAN-USB (PCAN_USBBUS1)  Device=PEAK-System PCAN-USB (PCAN_USBBUS1)  ObjConstructor=canChannel('PEAK-System', 'PCAN_USBBUS1')  EnablePeriodicTransmit=on  MessagePeriod=0.005
  CAN Transmit6 : canlib/CAN Transmit  BlockHandle=6076.0004  DeviceMenu=PEAK-System PCAN-USB (PCAN_USBBUS1)  Device=PEAK-System PCAN-USB (PCAN_USBBUS1)  ObjConstructor=canChannel('PEAK-System', 'PCAN_USBBUS1')  EnablePeriodicTransmit=on  MessagePeriod=0.005
  CAN Transmit7 : canlib/CAN Transmit  BlockHandle=6599.0004  DeviceMenu=PEAK-System PCAN-USB (PCAN_USBBUS1)  Device=PEAK-System PCAN-USB (PCAN_USBBUS1)  ObjConstructor=canChannel('PEAK-System', 'PCAN_USBBUS1')  EnablePeriodicTransmit=on  MessagePeriod=0.005
  CAN Transmit8 : canlib/CAN Transmit  BlockHandle=7059.0005  DeviceMenu=PEAK-System PCAN-USB (PCAN_USBBUS1)  Device=PEAK-System PCAN-USB (PCAN_USBBUS1)  ObjConstructor=canChannel('PEAK-System', 'PCAN_USBBUS1')  EnablePeriodicTransmit=on  MessagePeriod=0.005
  CAN Transmit9 : canlib/CAN Transmit  BlockHandle=7063.0002  DeviceMenu=PEAK-System PCAN-USB (PCAN_USBBUS1)  Device=PEAK-System PCAN-USB (PCAN_USBBUS1)  ObjConstructor=canChannel('PEAK-System', 'PCAN_USBBUS1')  EnablePeriodicTransmit=on  MessagePeriod=0.005
  wires:
  SensorInput/1 -> Bus Selector/1
  Bus Selector/1 -> CAN Pack1/1  "<Input_throttle>"
  CAN Pack1/1 -> CAN Transmit4/1
  Bus Selector/2 -> CAN Pack2/1  "<Input_brake>"
  CAN Pack2/1 -> CAN Transmit5/1
  CAN Pack3/1 -> CAN Transmit6/1
  Bus Selector/3 -> CAN Pack3/1  "<Input_steering>"
  Bus Selector/4 -> CAN Pack4/1  "<V_x>"
  CAN Pack4/1 -> CAN Transmit7/1
  Bus Selector/5 -> CAN Pack5/1  "<V_y>"
  Bus Selector/6 -> CAN Pack7/1  "<r>"
  Bus Selector/7 -> CAN Pack8/1  "<ay>"
  Bus Selector/8 -> CAN Pack10/1  "<ax>"
  Bus Selector/9 -> CAN Pack9/1  "<roll_angle>"
  Bus Selector/10 -> CAN Pack11/1  "<roll_rate>"
  Bus Selector/11 -> CAN Pack12/1  "<RPM_FL>"
  Bus Selector/12 -> CAN Pack13/1  "<RPM_FR>"
  CAN Pack16/1 -> CAN Transmit18/1
  Bus Selector/13 -> CAN Pack14/1  "<RPM_RL>"
  Bus Selector/14 -> CAN Pack15/1  "<RPM_RR>"
  Bus Selector/15 -> CAN Pack16/1  "<KERS_pos>"
  Fz_CM/1 -> Bus Selector1/1
  CAN Pack6/1 -> CAN Transmit1/1
  CAN Pack17/1 -> CAN Transmit/1
  CAN Pack18/1 -> CAN Transmit3/1
  CAN Pack19/1 -> CAN Transmit2/1
  Bus Selector1/1 -> CAN Pack17/1  "<FL>"
  Bus Selector1/2 -> CAN Pack6/1  "<FR>"
  Bus Selector1/4 -> CAN Pack18/1  "<RR>"
  Bus Selector1/3 -> CAN Pack19/1  "<RL>"
  CAN Pack20/1 -> CAN Transmit19/1

== system UnusedModels/Coasting KERS at 0 torque request ==
  states : Inport
  MATLAB Function : MATLAB Function  TreatAsAtomicUnit=on
  active : Outport
  Ti_coast : Outport  Port=2
  wires:
  states/1 -> MATLAB Function/1(states)
  MATLAB Function/1(active) -> active/1
  MATLAB Function/2(Ti_coast) -> Ti_coast/1

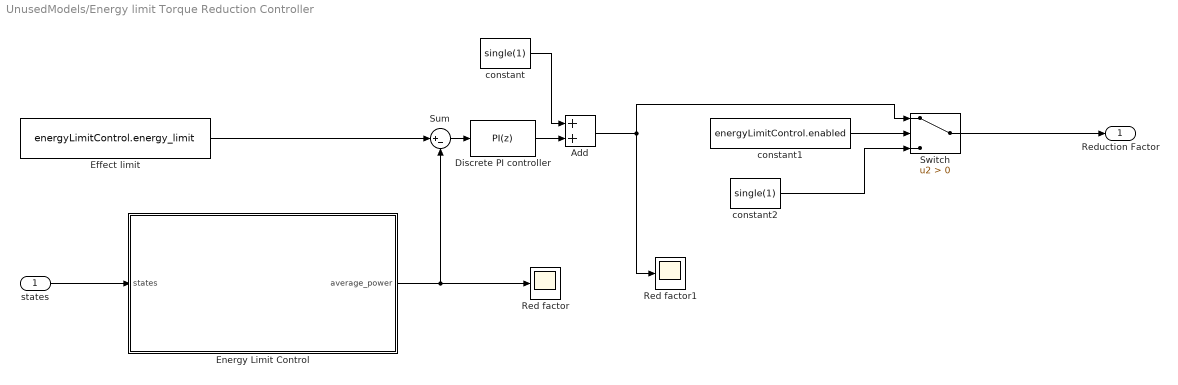
== system UnusedModels/Energy limit Torque Reduction Controller ==
  states : Inport
  Add : Sum
  Discrete PI controller : simulink/Continuous/PID Controller  Controller=PI  TimeDomain=Discrete-time  SampleTime=-1  IntegratorMethod=Forward Euler  FilterMethod=Forward Euler  Form=Parallel  UseFilter=on  ControllerParametersSource=internal  P=energyLimitControl.Kp;  I=energyLimitControl.Ki  D=0  N=100  InitialConditionSource=internal  InitialConditionForIntegrator=0  InitialConditionForFilter=0  ExternalReset=none  LimitOutput=on  UpperSaturationLimit=energyLimitControl.upper_sat_limit;  LowerSaturationLimit=energyLimitControl.lower_sat_limit;  LinearizeAsGain=off  AntiWindupMode=clamping  Kb=settings.Kb_EL;  TrackingMode=off  Kt=1  PParamMin=[]  PParamMax=[]  IParamMin=[]  IParamMax=[]  DParamMin=[]  DParamMax=[]  NParamMin=[]  NParamMax=[]  KbParamMin=[]  KbParamMax=[]  KtParamMin=[]  KtParamMax=[]  POutMin=[]  POutMax=[]  IOutMin=[]  IOutMax=[]  DOutMin=[]  DOutMax=[]  NOutMin=[]  NOutMax=[]  KbOutMin=[]  KbOutMax=[]  KtOutMin=[]  KtOutMax=[]  IntegratorOutMin=[]  IntegratorOutMax=[]  FilterOutMin=[]  FilterOutMax=[]  SumOutMin=[]  SumOutMax=[]  SumI1OutMin=[]  SumI1OutMax=[]  SumI2OutMin=[]  SumI2OutMax=[]  SumI3OutMin=[]  SumI3OutMax=[]  SumDOutMin=[]  SumDOutMax=[]  SaturationOutMin=[]  SaturationOutMax=[]  IntegratorContinuousStateAttributes=''  IntegratorStateMustResolveToSignalObject=off  IntegratorRTWStateStorageClass=Auto  FilterContinuousStateAttributes=''  FilterStateMustResolveToSignalObject=off  FilterRTWStateStorageClass=Auto  DifferentiatorICPrevScaledInput=0  DifferentiatorOutMin=[]  DifferentiatorOutMax=[]
  "Effect limit " : Constant  Value=energyLimitControl.energy_limit
  Energy Limit Control : MATLAB Function  TreatAsAtomicUnit=on
  Red factor : Scope
      settings: ShowLegends=on  TimeRange=10  YMin=0.011  YMax=0.023  SaveName=ScopeData38
  Red factor1 : Scope
      settings: ShowLegends=on  TimeRange=10  YMin=0.011  YMax=0.023  SaveName=ScopeData44
  Sum : Sum  Inputs=|+-
  Switch : Switch  Criteria=u2 > Threshold
  constant : Constant  Value=single(1)
  constant1 : Constant  Value=energyLimitControl.enabled
  constant2 : Constant  Value=single(1)
  Reduction Factor : Outport
  wires:
  Energy Limit Control/1(average_power) -> Sum/2, Red factor/1
  "Effect limit "/1 -> Sum/1
  Sum/1 -> Discrete PI controller/1
  Discrete PI controller/1 -> Add/2
  constant/1 -> Add/1
  Add/1 -> Switch/1, Red factor1/1
  states/1 -> Energy Limit Control/1(states)
  constant1/1 -> Switch/2
  constant2/1 -> Switch/3
  Switch/1 -> Reduction Factor/1

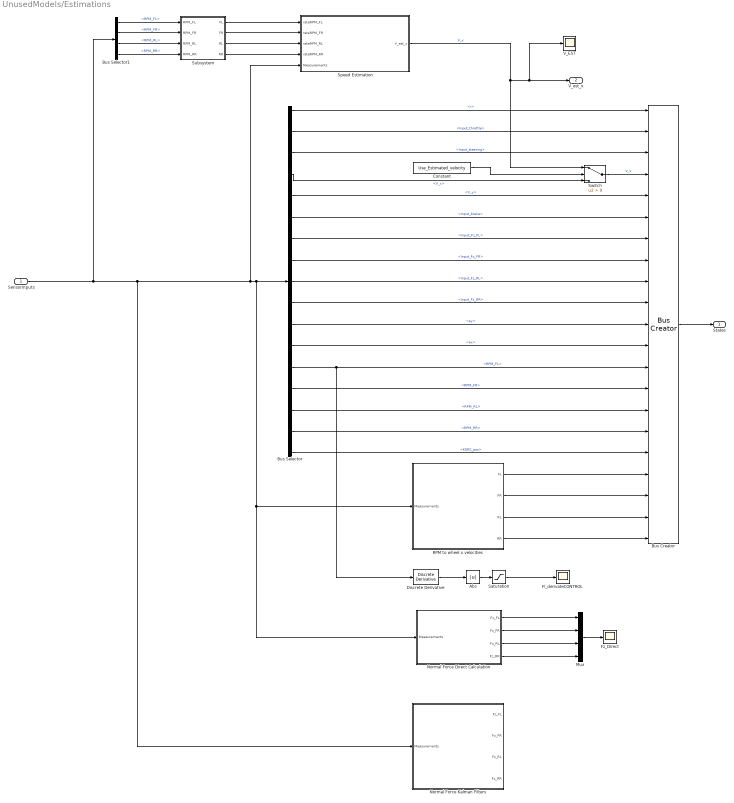
== system UnusedModels/Estimations  ==
  "SensorInputs " : Inport
  Abs : Abs
  Bus Creator : BusCreator  Inputs=21  OutDataTypeStr=Bus: States  NonVirtualBus=on
      settings: InheritFromInputs=off
  Bus Selector : BusSelector  OutputSignals=r,Input_throttle,Input_steering,V_x,V_y,Input_brake,Input_Fz_FL,Input_Fz_FR,Input_Fz_RL,Input_Fz_RR,ay,ax,RPM_FL,RPM_FR,RPM_RL,RPM_RR,KERS_pos
  Bus Selector1 : BusSelector  OutputSignals=RPM_FL,RPM_FR,RPM_RL,RPM_RR
  Constant : Constant  Value=Use_Estimated_velocity
  Discrete Derivative : simulink/Discrete/Discrete Derivative  gainval=1.0  ICPrevScaledInput=0.0  InputProcessing=Inherited  OutMin=[]  OutMax=[]  OutDataType=fixdt(1, 16)  OutScaling=2^-10  DoSatur=off
  Fl_derivateCONTROL : Scope
      settings: ShowLegends=on  TimeRange=3.722  YMin=0  YMax=10000  SaveName=ScopeData70
  Fz_Direct : Scope
      settings: ShowLegends=on  TimeRange=2.924148098991849  YMin=0  YMax=1600  SaveName=ScopeData58
  Mux : Mux
  Normal Force Direct Calculation : Subsystem
  Normal Force Kalman Filters : Subsystem
  RPM to wheel x velocities : Subsystem
  Saturation : Saturate  UpperLimit=50000
  Speed Estimation : Subsystem
  Subsystem : Subsystem
  Switch : Switch  Criteria=u2 > Threshold
  "V_EST " : Scope
      settings: ShowLegends=on  TimeRange=0.0008904109589041094  YMin=11.052  YMax=11.0585  SaveName=ScopeData37
  States : Outport
  V_est_x : Outport  Port=2
  wires:
  Bus Selector/3 -> Bus Creator/3  "<Input_steering>"
  Bus Creator/1 -> States/1
  "SensorInputs "/1 -> Bus Selector1/1, Bus Selector/1, Normal Force Direct Calculation/1(Measurements), RPM to wheel x velocities/1(Measurements), Speed Estimation/5(Measurements), Normal Force Kalman Filters/1(Measurements)
  Bus Selector/2 -> Bus Creator/2  "<Input_throttle>"
  Bus Selector/1 -> Bus Creator/1  "<r>"
  Bus Selector/4 -> Switch/3  "<V_x>"
  Bus Selector/5 -> Bus Creator/5  "<V_y>"
  Bus Selector/6 -> Bus Creator/6  "<Input_brake>"
  Bus Selector/11 -> Bus Creator/11  "<ay>"
  Bus Selector/12 -> Bus Creator/12  "<ax>"
  Bus Selector/13 -> Discrete Derivative/1, Bus Creator/13  "<RPM_FL>"
  Bus Selector/14 -> Bus Creator/14  "<RPM_FR>"
  Bus Selector/15 -> Bus Creator/15  "<RPM_RL>"
  Bus Selector/16 -> Bus Creator/16  "<RPM_RR>"
  Bus Selector/17 -> Bus Creator/17  "<KERS_pos>"
  RPM to wheel x velocities/1(FL) -> Bus Creator/18
  RPM to wheel x velocities/2(FR) -> Bus Creator/19
  RPM to wheel x velocities/3(RL) -> Bus Creator/20
  RPM to wheel x velocities/4(RR) -> Bus Creator/21
  Speed Estimation/1(V_est_x) -> Switch/1, V_est_x/1, "V_EST "/1  "V_x"
  Mux/1 -> Fz_Direct/1
  Normal Force Direct Calculation/1(Fz_FL) -> Mux/1
  Normal Force Direct Calculation/2(Fz_FR) -> Mux/2
  Normal Force Direct Calculation/3(Fz_RL) -> Mux/3
  Normal Force Direct Calculation/4(Fz_RR) -> Mux/4
  Switch/1 -> Bus Creator/4  "V_x"
  Constant/1 -> Switch/2
  Discrete Derivative/1 -> Abs/1
  Abs/1 -> Saturation/1
  Saturation/1 -> Fl_derivateCONTROL/1
  Bus Selector1/2 -> Subsystem/2(RPM_FR)  "<RPM_FR>"
  Bus Selector1/1 -> Subsystem/1(RPM_FL)  "<RPM_FL>"
  Bus Selector1/3 -> Subsystem/3(RPM_RL)  "<RPM_RL>"
  Bus Selector1/4 -> Subsystem/4(RPM_RR)  "<RPM_RR>"
  Bus Selector/7 -> Bus Creator/7  "<Input_Fz_FL>"
  Bus Selector/8 -> Bus Creator/8  "<Input_Fz_FR>"
  Bus Selector/9 -> Bus Creator/9  "<Input_Fz_RL>"
  Bus Selector/10 -> Bus Creator/10  "<Input_Fz_RR>"
  Subsystem/1(FL) -> Speed Estimation/1(rateRPM_FL)
  Subsystem/2(FR) -> Speed Estimation/2(rateRPM_FR)
  Subsystem/3(RL) -> Speed Estimation/3(rateRPM_RL)
  Subsystem/4(RR) -> Speed Estimation/4(rateRPM_RR)

== system UnusedModels/Function-Call Subsystem ==
  CAN_MSG : Inport
  function : TriggerPort  TriggerType=function-call
  CAN Unpack : canmsglib/CAN Unpack  MsgList=(none)  MsgName=INV_FL  MsgIDType=Standard (11-bit identifier)  MsgIdentifier=CAN_ID_INV_FL  MsgLength=6  SignalInfo=trq_pos$0$16$1$1$1$0$1$0$-Inf$Inf$#trq_neg$16$16$1$1$1$0$1$0$-Inf$Inf$#w_set$32$16$1$1$1$0$1$0$-Inf$Inf$#  NSignals=3  IDPort=off  TimestampPort=off  ErrorPort=off  RemotePort=off  LengthPort=off  StatusPort=off  StartBits=str2num('[int32(0);int32(16);int32(32)]')  SignalSizes=str2num('[int32(16);int32(16);int32(16)]')  ByteOrders=str2num('[int32(1);int32(1);int32(1)]')  DataTypes=str2num('[int32(1);int32(1);int32(1)]')  MultiplexTypes=str2num('[int32(1);int32(1);int32(1)]')  MultiplexValues=str2num('[double(0);double(0);double(0)]')  Factors=str2num('[double(1);double(1);double(1)]')  Offsets=str2num('[double(0);double(0);double(0)]')  Minimums=str2num('[double(-Inf);double(-Inf);double(-Inf)]')  Maximums=str2num('[double(Inf);double(Inf);double(Inf)]')
  MATLAB Function : MATLAB Function  TreatAsAtomicUnit=on
  Write CM Dict1 : CarMaker4SL/Write CM Dict  xname=Tlim_pos_FL  xsync=off
  Write CM Dict20 : CarMaker4SL/Write CM Dict  xname=Tlim_neg_FL  xsync=off
  Write CM Dict27 : CarMaker4SL/Write CM Dict  xname=w_set_FL  xsync=off
  wires:
  CAN_MSG/1 -> CAN Unpack/1
  CAN Unpack/2 -> MATLAB Function/2(trq_neg_16)
  CAN Unpack/3 -> MATLAB Function/3(w_set_16)
  CAN Unpack/1 -> MATLAB Function/1(trq_pos_16)
  MATLAB Function/1(trq_pos_f) -> Write CM Dict1/1
  MATLAB Function/2(trq_neg_f) -> Write CM Dict20/1
  MATLAB Function/3(w_set_f) -> Write CM Dict27/1

== system UnusedModels/Function-Call Subsystem1 ==
  CAN_MSG : Inport
  function : TriggerPort  TriggerType=function-call
  CAN Unpack1 : canmsglib/CAN Unpack  MsgList=(none)  MsgName=INV_FR  MsgIDType=Standard (11-bit identifier)  MsgIdentifier=CAN_ID_INV_FR  MsgLength=6  SignalInfo=trq_pos$0$16$1$1$1$0$1$0$-Inf$Inf$#trq_neg$16$16$1$1$1$0$1$0$-Inf$Inf$#w_set$32$16$1$1$1$0$1$0$-Inf$Inf$#  NSignals=3  IDPort=off  TimestampPort=off  ErrorPort=off  RemotePort=off  LengthPort=off  StatusPort=off  StartBits=str2num('[int32(0);int32(16);int32(32)]')  SignalSizes=str2num('[int32(16);int32(16);int32(16)]')  ByteOrders=str2num('[int32(1);int32(1);int32(1)]')  DataTypes=str2num('[int32(1);int32(1);int32(1)]')  MultiplexTypes=str2num('[int32(1);int32(1);int32(1)]')  MultiplexValues=str2num('[double(0);double(0);double(0)]')  Factors=str2num('[double(1);double(1);double(1)]')  Offsets=str2num('[double(0);double(0);double(0)]')  Minimums=str2num('[double(-Inf);double(-Inf);double(-Inf)]')  Maximums=str2num('[double(Inf);double(Inf);double(Inf)]')
  MATLAB Function1 : MATLAB Function  TreatAsAtomicUnit=on
  Write CM Dict11 : CarMaker4SL/Write CM Dict  xname=Tlim_neg_FR  xsync=off
  Write CM Dict13 : CarMaker4SL/Write CM Dict  xname=w_set_FR  xsync=off
  Write CM Dict2 : CarMaker4SL/Write CM Dict  xname=Tlim_pos_FR  xsync=off
  wires:
  CAN Unpack1/2 -> MATLAB Function1/2(trq_neg_16)
  CAN Unpack1/1 -> MATLAB Function1/1(trq_pos_16)
  CAN Unpack1/3 -> MATLAB Function1/3(w_set_16)
  MATLAB Function1/1(trq_pos_f) -> Write CM Dict2/1
  MATLAB Function1/2(trq_neg_f) -> Write CM Dict11/1
  MATLAB Function1/3(w_set_f) -> Write CM Dict13/1
  CAN_MSG/1 -> CAN Unpack1/1

== system UnusedModels/Function-Call Subsystem2 ==
  CAN_MSG : Inport
  function : TriggerPort  TriggerType=function-call
  CAN Unpack2 : canmsglib/CAN Unpack  MsgList=(none)  MsgName=INV_RL  MsgIDType=Standard (11-bit identifier)  MsgIdentifier=CAN_ID_INV_RL  MsgLength=6  SignalInfo=trq_pos$0$16$1$1$1$0$1$0$-Inf$Inf$#trq_neg$16$16$1$1$1$0$1$0$-Inf$Inf$#w_set$32$16$1$1$1$0$1$0$-Inf$Inf$#  NSignals=3  IDPort=off  TimestampPort=off  ErrorPort=off  RemotePort=off  LengthPort=off  StatusPort=off  StartBits=str2num('[int32(0);int32(16);int32(32)]')  SignalSizes=str2num('[int32(16);int32(16);int32(16)]')  ByteOrders=str2num('[int32(1);int32(1);int32(1)]')  DataTypes=str2num('[int32(1);int32(1);int32(1)]')  MultiplexTypes=str2num('[int32(1);int32(1);int32(1)]')  MultiplexValues=str2num('[double(0);double(0);double(0)]')  Factors=str2num('[double(1);double(1);double(1)]')  Offsets=str2num('[double(0);double(0);double(0)]')  Minimums=str2num('[double(-Inf);double(-Inf);double(-Inf)]')  Maximums=str2num('[double(Inf);double(Inf);double(Inf)]')
  MATLAB Function2 : MATLAB Function  TreatAsAtomicUnit=on
  Write CM Dict15 : CarMaker4SL/Write CM Dict  xname=Tlim_neg_RL  xsync=off
  Write CM Dict16 : CarMaker4SL/Write CM Dict  xname=w_set_RL  xsync=off
  Write CM Dict3 : CarMaker4SL/Write CM Dict  xname=Tlim_pos_RL  xsync=off
  wires:
  CAN Unpack2/1 -> MATLAB Function2/1(trq_pos_16)
  CAN Unpack2/2 -> MATLAB Function2/2(trq_neg_16)
  CAN Unpack2/3 -> MATLAB Function2/3(w_set_16)
  MATLAB Function2/3(w_set_f) -> Write CM Dict16/1
  MATLAB Function2/2(trq_neg_f) -> Write CM Dict15/1
  MATLAB Function2/1(trq_pos_f) -> Write CM Dict3/1
  CAN_MSG/1 -> CAN Unpack2/1

== system UnusedModels/Function-Call Subsystem3 ==
  CAN_MSG : Inport
  function : TriggerPort  TriggerType=function-call
  CAN Unpack3 : canmsglib/CAN Unpack  MsgList=(none)  MsgName=INV_RR  MsgIDType=Standard (11-bit identifier)  MsgIdentifier=CAN_ID_INV_RR  MsgLength=6  SignalInfo=trq_pos$0$16$1$1$1$0$1$0$-Inf$Inf$#trq_neg$16$16$1$1$1$0$1$0$-Inf$Inf$#w_set$32$16$1$1$1$0$1$0$-Inf$Inf$#  NSignals=3  IDPort=off  TimestampPort=off  ErrorPort=off  RemotePort=off  LengthPort=off  StatusPort=off  StartBits=str2num('[int32(0);int32(16);int32(32)]')  SignalSizes=str2num('[int32(16);int32(16);int32(16)]')  ByteOrders=str2num('[int32(1);int32(1);int32(1)]')  DataTypes=str2num('[int32(1);int32(1);int32(1)]')  MultiplexTypes=str2num('[int32(1);int32(1);int32(1)]')  MultiplexValues=str2num('[double(0);double(0);double(0)]')  Factors=str2num('[double(1);double(1);double(1)]')  Offsets=str2num('[double(0);double(0);double(0)]')  Minimums=str2num('[double(-Inf);double(-Inf);double(-Inf)]')  Maximums=str2num('[double(Inf);double(Inf);double(Inf)]')
  MATLAB Function3 : MATLAB Function  TreatAsAtomicUnit=on
  Write CM Dict18 : CarMaker4SL/Write CM Dict  xname=Tlim_neg_RR  xsync=off
  Write CM Dict19 : CarMaker4SL/Write CM Dict  xname=w_set_RR  xsync=off
  Write CM Dict4 : CarMaker4SL/Write CM Dict  xname=Tlim_pos_RR  xsync=off
  wires:
  CAN Unpack3/1 -> MATLAB Function3/1(trq_pos_16)
  CAN Unpack3/2 -> MATLAB Function3/2(trq_neg_16)
  CAN Unpack3/3 -> MATLAB Function3/3(w_set_16)
  MATLAB Function3/3(w_set_f) -> Write CM Dict19/1
  MATLAB Function3/2(trq_neg_f) -> Write CM Dict18/1
  MATLAB Function3/1(trq_pos_f) -> Write CM Dict4/1
  CAN_MSG/1 -> CAN Unpack3/1
